simulink model "testing_stuff"  (R2023b)
settings: Solver=VariableStepAuto  StartTime=0.0  StopTime=10.0  RelTol=1e-3
values from neighbouring files (symbols this model uses):
  mask = [1 1 0 0 0 0]    [EJ3.m]
  OW_R2x2 = OW_T(1:2,1:2)    [EJ3.m]
  OW_T = transl(1,1,0)*trotz(pi/4)    [EJ3.m]
  q0 = [pi/2,-pi/2]    [EJ3.m]
  robot = SerialLink(L, 'tool', Tool)    [EJ3.m]
  WO_R2x2 = WO_T(1:2,1:2)    [EJ3.m]
  WO_T = trotz(-pi/4)*transl(-1,-1,0)    [EJ3.m]
undefined symbols (not defined in the file or in its folder): coriolis, fkine, friction, gravload, inertia, jacob0, subsref
libraries: roblocks x2, matrix_library x1
settings Model: Creator=alero  LastModifiedBy=alero

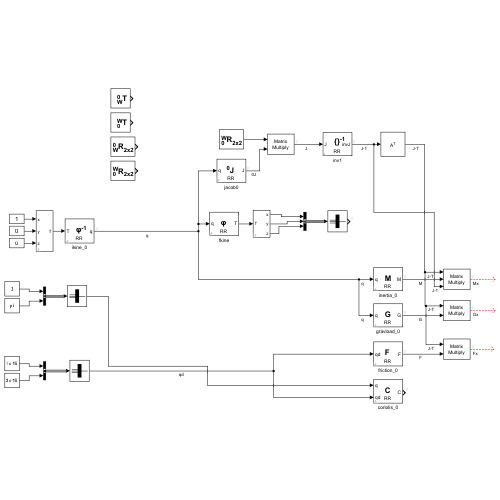
[thumbnail: Simulink's stored preview of the top-level diagram]
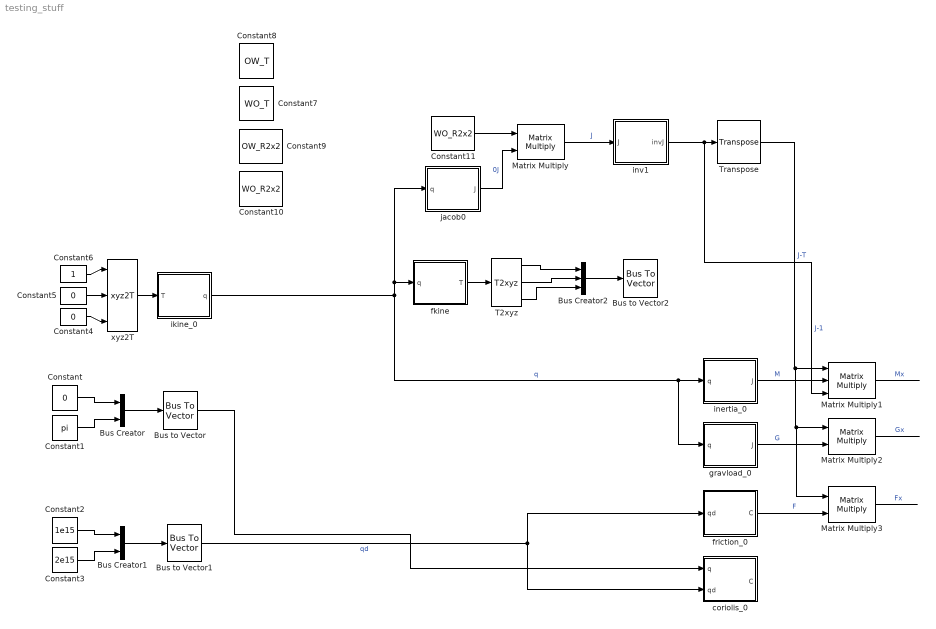
== system testing_stuff ==
  Bus Creator : BusCreator  Inputs=2
  Bus Creator1 : BusCreator  Inputs=2
  Bus Creator2 : BusCreator  Inputs=3
  Bus to Vector : BusToVector
  Bus to Vector1 : BusToVector
  Bus to Vector2 : BusToVector
  Constant : Constant  Value=0
  Constant1 : Constant  Value=pi
  Constant10 : Constant  Value=WO_R2x2  VectorParams1D=off
      mask Display:
      | text(0.1, 0.8, '\bf\fontsize{16}^W_0R_{2x2}', 'texmode', 'on', 'verticalAlignment', 'top', 'horizontalAlignment', 'left')
      | %text(0.45, 0.65, '\fontsize{10}0', 'texmode', 'on','verticalAlignment', 'bottom', 'horizontalAlignment', 'right')
  Constant11 : Constant  Value=WO_R2x2  VectorParams1D=off
      mask Display:
      | text(0.1, 0.8, '\bf\fontsize{16}^W_0R_{2x2}', 'texmode', 'on', 'verticalAlignment', 'top', 'horizontalAlignment', 'left')
      | %text(0.45, 0.65, '\fontsize{10}0', 'texmode', 'on','verticalAlignment', 'bottom', 'horizontalAlignment', 'right')
  Constant2 : Constant  Value=1e15
  Constant3 : Constant  Value=2e15
  Constant4 : Constant  Value=0
  Constant5 : Constant  Value=0
  Constant6 : Constant
  Constant7 : Constant  Value=WO_T  VectorParams1D=off
      mask Display:
      | text(0.35, 0.8, '\bf\fontsize{16}^W_0T', 'texmode', 'on', 'verticalAlignment', 'top', 'horizontalAlignment', 'left')
      | %text(0.45, 0.65, '\fontsize{10}0', 'texmode', 'on','verticalAlignment', 'bottom', 'horizontalAlignment', 'right')
  Constant8 : Constant  Value=OW_T  VectorParams1D=off
      mask Display:
      | text(0.35, 0.8, '\bf\fontsize{16}^0_WT', 'texmode', 'on', 'verticalAlignment', 'top', 'horizontalAlignment', 'left')
      | %text(0.45, 0.65, '\fontsize{10}0', 'texmode', 'on','verticalAlignment', 'bottom', 'horizontalAlignment', 'right')
  Constant9 : Constant  Value=OW_R2x2  VectorParams1D=off
      mask Display:
      | text(0.1, 0.8, '\bf\fontsize{16}^0_WR_{2x2}', 'texmode', 'on', 'verticalAlignment', 'top', 'horizontalAlignment', 'left')
      | %text(0.45, 0.65, '\fontsize{10}0', 'texmode', 'on','verticalAlignment', 'bottom', 'horizontalAlignment', 'right')
  Matrix Multiply : Product  Multiplication=Matrix(*)
  Matrix Multiply1 : Product  Inputs=3  Multiplication=Matrix(*)
  Matrix Multiply2 : Product  Multiplication=Matrix(*)
  Matrix Multiply3 : Product  Multiplication=Matrix(*)
  T2xyz : roblocks/Toolbox/T2xyz
  Transpose : matrix_library/Transpose
  coriolis_0 : Subsystem  mask{robot=robot}
      mask prompts: robot "Robot object"
      mask help: Robot Jacobian in world coordinates
      mask init:
      | if ~isempty(robot)
      |     n=robot.n;
      | end
      mask Help:
      | Jacobian matrix relating joint coordinate rates to end-effector spatial
      | velocity expressed in the world frame.
      | 
      | <b>Parameters::</b>
      | 
      | Robot (SerialLink class)  The N-axis robot object for which the Jacobian is
      |                           computed.
      | 
      | <b>Inputs::</b>
      | 
      | q (1xN) joint coordinates
      | 
      | <b>Outputs::</b>
      | 
      | J (6xN) the Jacobian matrix
      | 
      | <b>Notes::</b>
      | 
      | - A wrapper for the Toolbox method jacob0().
      mask Display:
      | text(0.4, 0.8, '\bf\fontsize{16}C', 'texmode', 'on', 'verticalAlignment', 'top', 'horizontalAlignment', 'left')
      | %text(0.45, 0.65, '\fontsize{10}0', 'texmode', 'on','verticalAlignment', 'bottom', 'horizontalAlignment', 'right')
      | if ~isempty(robot)
      |     text(0.5, 0.2, robot.name,  'horizontalAlignment', 'center')
      | end
      | port_label('input', 1, 'q')
      | port_label('output', 1, 'C')
      | port_label('input',2,'qd')
  fkine : Subsystem  mask{robot=robot}
      mask prompts: robot "Robot object"
      mask help: Robot forward kinematics.
      mask Help:
      | Compute homogeneous transform for robot end-effector given joint coordinates
      | 
      | 
      | <b>Parameters::</b>
      | 
      | Robot (SerialLink class)  The N-axis robot object for computing forward kinematics.
      | 
      | <b>Inputs::</b>
      | 
      | q (1xN) joint coordinates
      | 
      | <b>Outputs::</b>
      | 
      | T (4x4) the pose of the end effector as a homogeneous transformation
      | 
      | <b>Notes::</b>
      | 
      | - A wrapper for the Toolbox method fkine().
      mask Display:
      | text(0.4, 0.8, '\bf\fontsize{16}\phi', 'texmode', 'on', 'verticalAlignment', 'top', 'horizontalAlignment', 'left')
      | %text(0.45, 0.65, '\fontsize{10}0', 'texmode', 'on','verticalAlignment', 'bottom', 'horizontalAlignment', 'right')
      | if ~isempty(robot)
      |     text(0.5, 0.2, robot.name,  'horizontalAlignment', 'center')
      | end
      | port_label('input', 1, 'q')
      | port_label('output', 1, 'T')
  friction_0 : Subsystem  mask{robot=robot}
      mask prompts: robot "Robot object"
      mask help: Robot Jacobian in world coordinates
      mask init:
      | if ~isempty(robot)
      |     n=robot.n;
      | end
      mask Help:
      | Jacobian matrix relating joint coordinate rates to end-effector spatial
      | velocity expressed in the world frame.
      | 
      | <b>Parameters::</b>
      | 
      | Robot (SerialLink class)  The N-axis robot object for which the Jacobian is
      |                           computed.
      | 
      | <b>Inputs::</b>
      | 
      | q (1xN) joint coordinates
      | 
      | <b>Outputs::</b>
      | 
      | J (6xN) the Jacobian matrix
      | 
      | <b>Notes::</b>
      | 
      | - A wrapper for the Toolbox method jacob0().
      mask Display:
      | text(0.4, 0.8, '\bf\fontsize{16}F', 'texmode', 'on', 'verticalAlignment', 'top', 'horizontalAlignment', 'left')
      | %text(0.45, 0.65, '\fontsize{10}0', 'texmode', 'on','verticalAlignment', 'bottom', 'horizontalAlignment', 'right')
      | if ~isempty(robot)
      |     text(0.5, 0.2, robot.name,  'horizontalAlignment', 'center')
      | end
      | port_label('input', 1, 'qd')
      | port_label('output', 1, 'F')
  gravload_0 : Subsystem  mask{robot=robot}
      mask prompts: robot "Robot object"
      mask help: Robot Jacobian in world coordinates
      mask init:
      | if ~isempty(robot)
      |     n=robot.n;
      | end
      mask Help:
      | Jacobian matrix relating joint coordinate rates to end-effector spatial
      | velocity expressed in the world frame.
      | 
      | <b>Parameters::</b>
      | 
      | Robot (SerialLink class)  The N-axis robot object for which the Jacobian is
      |                           computed.
      | 
      | <b>Inputs::</b>
      | 
      | q (1xN) joint coordinates
      | 
      | <b>Outputs::</b>
      | 
      | J (6xN) the Jacobian matrix
      | 
      | <b>Notes::</b>
      | 
      | - A wrapper for the Toolbox method jacob0().
      mask Display:
      | text(0.4, 0.8, '\bf\fontsize{16}G', 'texmode', 'on', 'verticalAlignment', 'top', 'horizontalAlignment', 'left')
      | %text(0.45, 0.65, '\fontsize{10}0', 'texmode', 'on','verticalAlignment', 'bottom', 'horizontalAlignment', 'right')
      | if ~isempty(robot)
      |     text(0.5, 0.2, robot.name,  'horizontalAlignment', 'center')
      | end
      | port_label('input', 1, 'q')
      | port_label('output', 1, 'G')
  ikine_0 : Subsystem  mask{robot=robot, q0=q0, M=mask, pinv=off, options={}}
      mask prompts: robot "Robot object"; q0 "Initial q"; M "Mask vector"; pinv "Pseudo-inverse (pinv)"; options "Options (cell array)"
      mask help: Generalized numerical inverse kinematics
      mask init:
      | opt = options;
      | if pinv
      |     opt = [opt 'pinv'];
      | end
      | disp(opt)
      mask Help:
      | Compute joint coordinates for robot given end-effector pose.
      | 
      | 
      | <b>Parameters::</b>
      | 
      | Robot (SerialLink class)  The N-axis robot object for computing forward kinematics.
      | Initial q  (1xN)          Initial joint coordinates for solution
      | Mask vector (1x6)         Mask vector for underactuated manipulators.
      | Pseudo inverse (logical)  Enable option 'pinv'
      | Options                   Option value list to be passed to ikine()
      | 
      | <b>Inputs::</b>
      | 
      | T (4x4) the pose of the end effector as a homogeneous transformation
      | 
      | 
      | <b>Outputs::</b>
      | 
      | q (1xN) joint coordinates
      | 
      | <b>Notes::</b>
      | 
      | - A wrapper for the Toolbox method ikine().
      mask Display:
      | text(0.4, 0.8, '\bf\fontsize{16}\phi^{-1}', 'texmode', 'on', 'verticalAlignment', 'top', 'horizontalAlignment', 'left')
      | %text(0.45, 0.65, '\fontsize{10}0', 'texmode', 'on','verticalAlignment', 'bottom', 'horizontalAlignment', 'right')
      | if ~isempty(robot)
      |     text(0.5, 0.2, robot.name,  'horizontalAlignment', 'center')
      | end
      | port_label('input', 1, 'T')
      | port_label('output', 1, 'q')
  inertia_0 : Subsystem  mask{robot=robot}
      mask prompts: robot "Robot object"
      mask help: Robot Jacobian in world coordinates
      mask init:
      | if ~isempty(robot)
      |     n=robot.n;
      | end
      mask Help:
      | Jacobian matrix relating joint coordinate rates to end-effector spatial
      | velocity expressed in the world frame.
      | 
      | <b>Parameters::</b>
      | 
      | Robot (SerialLink class)  The N-axis robot object for which the Jacobian is
      |                           computed.
      | 
      | <b>Inputs::</b>
      | 
      | q (1xN) joint coordinates
      | 
      | <b>Outputs::</b>
      | 
      | J (6xN) the Jacobian matrix
      | 
      | <b>Notes::</b>
      | 
      | - A wrapper for the Toolbox method jacob0().
      mask Display:
      | text(0.4, 0.8, '\bf\fontsize{16}M', 'texmode', 'on', 'verticalAlignment', 'top', 'horizontalAlignment', 'left')
      | %text(0.45, 0.65, '\fontsize{10}0', 'texmode', 'on','verticalAlignment', 'bottom', 'horizontalAlignment', 'right')
      | if ~isempty(robot)
      |     text(0.5, 0.2, robot.name,  'horizontalAlignment', 'center')
      | end
      | port_label('input', 1, 'q')
      | port_label('output', 1, 'M')
  inv1 : Subsystem  mask{robot=robot}
      mask prompts: robot "Robot object"
      mask help: Robot Jacobian in world coordinates
      mask init:
      | if ~isempty(robot)
      |     n=robot.n;
      | end
      mask Help:
      | Jacobian matrix relating joint coordinate rates to end-effector spatial
      | velocity expressed in the world frame.
      | 
      | <b>Parameters::</b>
      | 
      | Robot (SerialLink class)  The N-axis robot object for which the Jacobian is
      |                           computed.
      | 
      | <b>Inputs::</b>
      | 
      | q (1xN) joint coordinates
      | 
      | <b>Outputs::</b>
      | 
      | J (6xN) the Jacobian matrix
      | 
      | <b>Notes::</b>
      | 
      | - A wrapper for the Toolbox method jacob0().
      mask Display:
      | text(0.4, 0.9, '\bf\fontsize{16}\{\}^{-1}', 'texmode', 'on', 'verticalAlignment', 'top', 'horizontalAlignment', 'left')
      | %text(0.45, 0.65, '\fontsize{10}0', 'texmode', 'on','verticalAlignment', 'bottom', 'horizontalAlignment', 'right')
      | if ~isempty(robot)
      |     text(0.5, 0.2, robot.name,  'horizontalAlignment', 'center')
      | end
      | port_label('input', 1, 'J')
      | port_label('output', 1, 'invJ')
  "jacob0 " : Subsystem  mask{robot=robot}
      mask prompts: robot "Robot object"
      mask help: Robot Jacobian in world coordinates
      mask init:
      | if ~isempty(robot)
      |     n=robot.n;
      | end
      mask Help:
      | Jacobian matrix relating joint coordinate rates to end-effector spatial
      | velocity expressed in the world frame.
      | 
      | <b>Parameters::</b>
      | 
      | Robot (SerialLink class)  The N-axis robot object for which the Jacobian is
      |                           computed.
      | 
      | <b>Inputs::</b>
      | 
      | q (1xN) joint coordinates
      | 
      | <b>Outputs::</b>
      | 
      | J (6xN) the Jacobian matrix
      | 
      | <b>Notes::</b>
      | 
      | - A wrapper for the Toolbox method jacob0().
      mask Display:
      | text(0.35, 0.8, '\bf\fontsize{16}^0J', 'texmode', 'on', 'verticalAlignment', 'top', 'horizontalAlignment', 'left')
      | %text(0.45, 0.65, '\fontsize{10}0', 'texmode', 'on','verticalAlignment', 'bottom', 'horizontalAlignment', 'right')
      | if ~isempty(robot)
      |     text(0.5, 0.2, robot.name,  'horizontalAlignment', 'center')
      | end
      | port_label('input', 1, 'q')
      | port_label('output', 1, 'J')
  xyz2T : roblocks/Toolbox/xyz2T
  wires:
  Bus Creator/1 -> Bus to Vector/1
  Constant/1 -> Bus Creator/1
  Constant1/1 -> Bus Creator/2
  Constant3/1 -> Bus Creator1/2
  Constant2/1 -> Bus Creator1/1
  Bus Creator1/1 -> Bus to Vector1/1
  Bus to Vector/1 -> coriolis_0/1(q)
  Bus to Vector1/1 -> coriolis_0/2(qd), friction_0/1(qd)  "qd"
  xyz2T/1 -> ikine_0/1(T)
  Constant4/1 -> xyz2T/3
  Constant5/1 -> xyz2T/2
  Constant6/1 -> xyz2T/1
  ikine_0/1(q) -> "jacob0 "/1(q), fkine/1(q), gravload_0/1(q), inertia_0/1(q)  "q"
  fkine/1(T) -> T2xyz/1
  T2xyz/2 -> Bus Creator2/2
  Bus Creator2/1 -> Bus to Vector2/1
  T2xyz/1 -> Bus Creator2/1
  T2xyz/3 -> Bus Creator2/3
  "jacob0 "/1(J) -> Matrix Multiply/2  "0J"
  Constant11/1 -> Matrix Multiply/1
  Matrix Multiply/1 -> inv1/1(J)  "J"
  inv1/1(invJ) -> Matrix Multiply1/3, Transpose/1  "J-1"
  Transpose/1 -> Matrix Multiply3/1, Matrix Multiply2/1, Matrix Multiply1/1  "J-T"
  inertia_0/1(J) -> Matrix Multiply1/2  "M"
  Matrix Multiply1/1 -> ?  "Mx"
  gravload_0/1(J) -> Matrix Multiply2/2  "G"
  Matrix Multiply2/1 -> ?  "Gx"
  Matrix Multiply3/1 -> ?  "Fx"
  friction_0/1(C) -> Matrix Multiply3/2  "F"

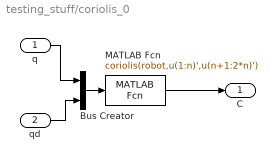
== system testing_stuff/coriolis_0 ==
  q : Inport
  qd : Inport  Port=2
  Bus Creator : BusCreator  Inputs=2
  MATLAB Fcn : MATLABFcn  MATLABFcn=coriolis(robot,u(1:n)',u(n+1:2*n)')  OutputDimensions=[robot.n robot.n]  Output1D=off
  C : Outport  VectorParamsAs1DForOutWhenUnconnected=off
  wires:
  MATLAB Fcn/1 -> C/1
  Bus Creator/1 -> MATLAB Fcn/1
  q/1 -> Bus Creator/1
  qd/1 -> Bus Creator/2

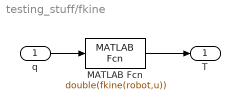
== system testing_stuff/fkine ==
  q : Inport
  MATLAB Fcn : MATLABFcn  MATLABFcn=double(fkine(robot,u))  OutputDimensions=[4 4]  Output1D=off
  T : Outport  VectorParamsAs1DForOutWhenUnconnected=off
  wires:
  q/1 -> MATLAB Fcn/1
  MATLAB Fcn/1 -> T/1

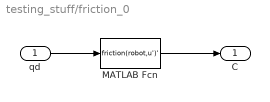
== system testing_stuff/friction_0 ==
  qd : Inport
  MATLAB Fcn : MATLABFcn  MATLABFcn=friction(robot,u')'  OutputDimensions=[robot.n 1]  Output1D=off
  C : Outport  VectorParamsAs1DForOutWhenUnconnected=off
  wires:
  MATLAB Fcn/1 -> C/1
  qd/1 -> MATLAB Fcn/1

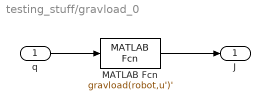
== system testing_stuff/gravload_0 ==
  q : Inport
  MATLAB Fcn : MATLABFcn  MATLABFcn=gravload(robot,u')'  OutputDimensions=[robot.n 1]  Output1D=off
  J : Outport  VectorParamsAs1DForOutWhenUnconnected=off
  wires:
  MATLAB Fcn/1 -> J/1
  q/1 -> MATLAB Fcn/1

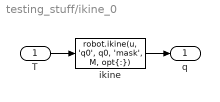
== system testing_stuff/ikine_0 ==
  T : Inport
  ikine : MATLABFcn  MATLABFcn=robot.ikine(u, 'q0', q0, 'mask', M, opt{:})
  q : Outport  VectorParamsAs1DForOutWhenUnconnected=off
  wires:
  ikine/1 -> q/1
  T/1 -> ikine/1

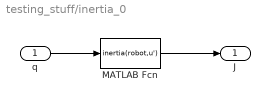
== system testing_stuff/inertia_0 ==
  q : Inport
  MATLAB Fcn : MATLABFcn  MATLABFcn=inertia(robot,u')  OutputDimensions=[robot.n robot.n]  Output1D=off
  J : Outport  VectorParamsAs1DForOutWhenUnconnected=off
  wires:
  MATLAB Fcn/1 -> J/1
  q/1 -> MATLAB Fcn/1

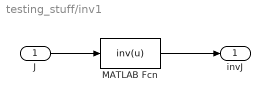
== system testing_stuff/inv1 ==
  J : Inport
  MATLAB Fcn : MATLABFcn  MATLABFcn=inv(u)  OutputDimensions=[n n]  Output1D=off
  invJ : Outport  VectorParamsAs1DForOutWhenUnconnected=off
  wires:
  MATLAB Fcn/1 -> invJ/1
  J/1 -> MATLAB Fcn/1

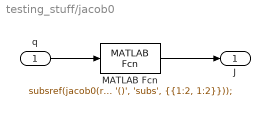
== system testing_stuff/jacob0  ==
  q : Inport
  MATLAB Fcn : MATLABFcn  MATLABFcn=subsref(jacob0(robot,u), struct('type', '()', 'subs', {{1:2, 1:2}}));  OutputDimensions=[n n]  Output1D=off
  J : Outport  VectorParamsAs1DForOutWhenUnconnected=off
  wires:
  MATLAB Fcn/1 -> J/1
  q/1 -> MATLAB Fcn/1
